simulink model "EnergyHub_V5_inf_buffer"  (R2024b)
settings: Solver=VariableStepAuto  StartTime=0  StopTime=31536000  MaxStep=1  RelTol=1e-3
values from neighbouring files (symbols this model uses):
  BatteryVNom = 51.2    [EdgeCases.m]    (also in MultipleModelTesting.m; setup_V3.m; setup_V5.m)
  ElectrolyserBoP = 80    [EdgeCases.m]    (also in setup_V3.m; setup_V5.m)
  ElectrolyserHoldTime = 25 * 60    (= 1500)    [EdgeCases.m]    (also in setup_V3.m; setup_V5.m)
  ElectrolyserHyFlow = 510    [EdgeCases.m]    (also in setup_V3.m; setup_V5.m)
  ElectrolyserPower = 2450    [EdgeCases.m]    (also in setup_V3.m = 2450/2:2450/2:2450*1.5; setup_V5.m)
  ElectrolyserRampDownTime = 30 * 60    (= 1800)    [EdgeCases.m]    (also in setup_V3.m; setup_V5.m)
  ElectrolyserRampUpTime = 10 * 60    (= 600)    [EdgeCases.m]    (also in setup_V3.m; setup_V5.m)
  ElectrolyserWarming = 260    [EdgeCases.m]    (also in setup_V3.m; setup_V5.m)
  ElectrolyserWarmingTime = 12 * 60    (= 720)    [EdgeCases.m]    (also in setup_V3.m; setup_V5.m)
  EMSElecStartHr = 14    [EdgeCases.m]    (also in setup_V3.m = 12:0.5:15; setup_V5.m)
  EMSElecStartSoC = 70    [EdgeCases.m]    (also in setup_V3.m = 70:5:80; setup_V5.m)
  EMSElecStopSoC = 65    [EdgeCases.m]    (also in setup_V3.m = 50:5:65; setup_V5.m)
  EMSFCSoCThresholds = [140, 150, 160, 170, 180]    [EdgeCases.m]    (also in setup_V3.m = [13, 14, 15, 16, 17]; setup_V5.m)
  EMSFCStartSoC = 15    [EdgeCases.m]    (also in MultipleModelTesting.m; setup_V3.m = 25; setup_V5.m)
  EMSFCStopSoC = 70    [EdgeCases.m]    (also in MultipleModelTesting.m; setup_V3.m = 90; setup_V5.m)
  EMSFCTimeThresholds = [113, 114, 115, 116, 117]    [EdgeCases.m]    (also in setup_V3.m = [40, 50, 60, 70, 80]; setup_V5.m)
  FuelCellAirBlower = 6.4*33.9    (= 216.96)    [EdgeCases.m]    (also in setup_V3.m; setup_V5.m)
  FuelCellBoP = 155    [EdgeCases.m]    (also in setup_V3.m; setup_V5.m)
  FuelCellHyFlow = 24    [EdgeCases.m]    (also in setup_V3.m = 31.7333333333; setup_V5.m)
  FuelCellPower = 2380    [EdgeCases.m]    (also in setup_V3.m = 1.2e3:300:1.8e3; setup_V5.m)
  FuelCellRampDown = 60    [EdgeCases.m]    (also in setup_V3.m; setup_V5.m)
  FuelCellRampTime1 = 40    [EdgeCases.m]    (also in setup_V3.m; setup_V5.m)
  FuelCellRampTime2 = 18*60    (= 1080)    [EdgeCases.m]    (also in setup_V3.m; setup_V5.m)
  FuelCellStartPower = 580    [EdgeCases.m]    (also in setup_V3.m; setup_V5.m)
  GridExtra = 0    [EdgeCases.m]    (also in setup_V3.m; setup_V5.m = 50)
  HydrogenCapacity = 70    [EdgeCases.m]    (also in setup_V3.m = 48; setup_V5.m)
  MinSoCGrid = EMSFCStartSoC-5    (= 10)    [EdgeCases.m]    (also in MultipleModelTesting.m; setup_V5.m)
  SolarPanels = 21    [EdgeCases.m]    (also in MultipleModelTesting.m = 12; setup_V3.m = 12:3:18; setup_V5.m = 18)
  SummerBase = 80    [EdgeCases.m]    (also in setup_V3.m; setup_V5.m)
  WinterBase = 235    [EdgeCases.m]    (also in setup_V3.m; setup_V5.m)
undefined symbols (not defined in the file or in its folder): Ion, Lithium
libraries: spsACVoltageSourceLib x3, spsBatteryLib x1, spsControlledCurrentSourceLib x1, sps_lib x1, simulink x1, spsGroundLib x1, spsPower3phInstantaneousLib x1, spsThreePhaseDynamicLoadLib x1, spsThreePhaseVIMeasurementLib x1
(part 1 of 2)
settings Model: Creator=daans  LastModifiedBy=daan
settings RTWCC: GPUComputeCapability=3.5

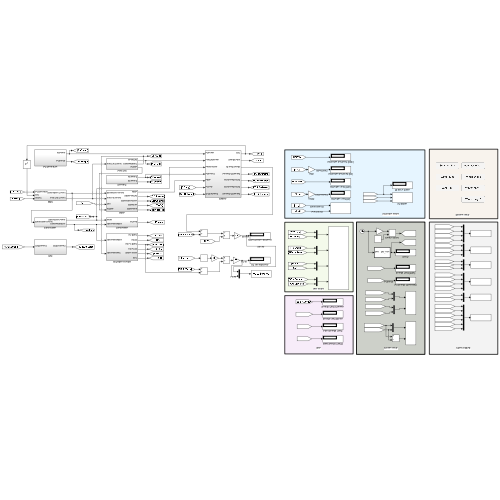
[thumbnail: Simulink's stored preview of the top-level diagram]
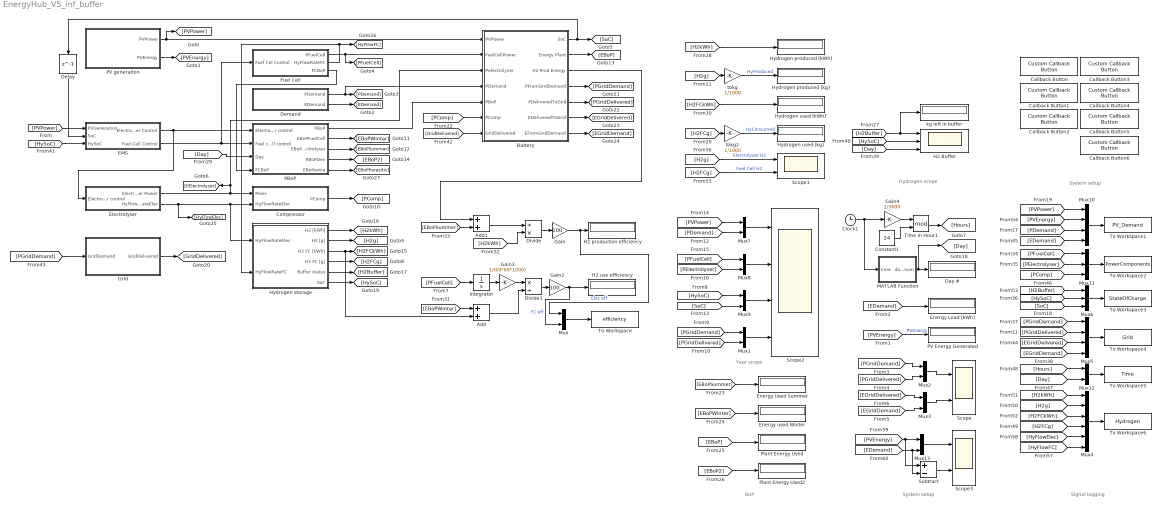
== system EnergyHub_V5_inf_buffer ==
  note: BoP
  note: System setup
  note: Year scope
  note: Hydrogen scope
  note: System setup
  note: Signal logging
  Add : Sum
  Add1 : Sum
  Battery : Subsystem
  Callback Button : CustomCallbackButton  Configuration="{\"components\":[{\"name\":\"BackgroundImageComponent\",\"settings\":{\"image\":{\"size\":[0,0],\"src\":\"default\",\"srcOrientation\":\"Right\"},\"position\":[0,0,1,1]}},{\"name\":\"ButtonStateComponent\",\"settings\":{\"buttonType\":\"momentary\",\"clickFcn\":\"% Define your start and stop time values\\nstartTime = 75*24*60*60;  % Example start time\\nstopTime = 289*24*60*60;   % Example stop time\\n\\n% Set the simulation start and stop time\\nset_param(gcs, 'StartTime', num2str(startTime));\\nset_param(gcs, 'StopTime', num2str(stopTime));\\n\\n% Optionally, start the simulation (if you want the button to trigger simulation)\\nset_param(gcs, 'SimulationCommand', 'start');\",\"onValue\":1,\"position\":[0,0,1,1],\"pressDelay\":\"500\",\"pressFcn\":\"\",\"repeatInterval\":\"0\",\"states\":[{\"horizontalAlignment\":\"center\",\"image\":{\"position\":[0,0,1,1],\"size\":[1,1],\"src\":\"default\",\"srcOrientation\":\"Right\"},\"label\":{\"color\":[0.01176470588,0.01176470588,0.01176470588,1],\"icon\":{\"size\":[0,0],\"src\":\"default\",\"srcOrientation\":\"Right\"},\"iconOffset\":0,\"iconPlacement\":\"left\",\"opacity\":1,\"show\":true,\"text\":{\"content\":\"Summer Sim\",\"font\":\"Helvetica\"}},\"labelOffset\":[0,0],\"verticalAlignment\":\"middle\"},{\"horizontalAlignment\":\"center\",\"image\":{\"position\":[0,0,1,1],\"size\":[1,1],\"src\":\"default\",\"srcOrientation\":\"Right\"},\"label\":{\"color\":[0.01176470588,0.01176470588,0.01176470588,1],\"icon\":{\"size\":[0,0],\"src\":\"default\",\"srcOrientation\":\"Right\"},\"iconOffset\":0,\"iconPlacement\":\"left\",\"opacity\":1,\"show\":true,\"text\":{\"content\":\"Summer Sim\",\"font\":\"Helvetica\"}},\"labelOffset\":[0,0],\"verticalAlignment\":\"middle\"},{\"horizontalAlignment\":\"center\",\"image\":{\"position\":[0,0,1,1],\"size\":[1,1],\"src\":\"default\",\"srcOrientation\":\"Right\"},\"label\":{\"color\":[0.01176470588,0.01176470588,0.01176470588,1],\"icon\":{\"size\":[0,0],\"src\":\"default\",\"srcOrientation\":\"Right\"},\"iconOffset\":0,\"iconPlacement\":\"left\",\"opacity\":1,\"show\":true,\"text\":{\"content\":\"Summer Sim\",\"font\":\"Helvetica\"}},\"labelOffset\":[0,0],\"verticalAlignment\":\"middle\"},{\"horizontalAlignment\":\"center\",\"image\":{\"position\":[0,0,1,1],\"size\":[1,1],\"src\":\"default\",\"srcOrientation\":\"Right\"},\"label\":{\"color\":[0.01176470588,0.01176470588,0.01176470588,1],\"icon\":{\"size\":[0,0],\"src\":\"default\",\"srcOrientation\":\"Right\"},\"iconOffset\":0,\"iconPlacement\":\"left\",\"opacity\":1,\"show\":true,\"text\":{\"content\":\"Summer Sim\",\"font\":\"Helvetica\"}},\"labelOffset\":[0,0],\"verticalAlignment\":\"middle\"}]}},{\"name\":\"ForegroundImageComponent\",\"settings\":{\"image\":{\"size\":[0,0],\"src\":\"default\",\"srcOrientation\":\"Right\"},\"isForeground\":1,\"position\":[0,0,1,1]}}],\"settings\":{\"BindingType\":\"standalone\",\"backgroundColor\":[244,244,244,1],\"backgroundOffset\":0.2,\"backgroundOpacity\":1,\"fixedAspectRatio\":\"off\",\"foregroundColor\":[0.01176470588,0.01176470588,0.01176470588,1],\"migratedFromLegacy\":true,\"useBackgroundColor\":true,\"variant\":\"callback\",\"version\":\"R2023a\"},\"type\":\"Button\"}"  CustomBackgroundColor="{\"color\":[0.9568627451,0.9568627451,0.9568627451],\"show\":true}"
  Callback Button1 : CustomCallbackButton  Configuration="{\"components\":[{\"name\":\"BackgroundImageComponent\",\"settings\":{\"image\":{\"size\":[0,0],\"src\":\"default\",\"srcOrientation\":\"Right\"},\"position\":[0,0,1,1]}},{\"name\":\"ButtonStateComponent\",\"settings\":{\"buttonType\":\"momentary\",\"clickFcn\":\"% Define your start and stop time values\\nstartTime = 19*24*60*60;  % Example start time\\nstopTime = 20*24*60*60;   % Example stop time\\n\\n% Set the simulation start and stop time\\nset_param(gcs, 'StartTime', num2str(startTime));\\nset_param(gcs, 'StopTime', num2str(stopTime));\\n\\n% Optionally, start the simulation (if you want the button to trigger simulation)\\nset_param(gcs, 'SimulationCommand', 'start');\",\"onValue\":1,\"position\":[0,0,1,1],\"pressDelay\":\"500\",\"pressFcn\":\"\",\"repeatInterval\":\"0\",\"states\":[{\"horizontalAlignment\":\"center\",\"image\":{\"position\":[0,0,1,1],\"size\":[1,1],\"src\":\"default\",\"srcOrientation\":\"Right\"},\"label\":{\"color\":[0.01176470588,0.01176470588,0.01176470588,1],\"icon\":{\"size\":[0,0],\"src\":\"default\",\"srcOrientation\":\"Right\"},\"iconOffset\":0,\"iconPlacement\":\"left\",\"opacity\":1,\"show\":true,\"text\":{\"content\":\"Winter Sim\",\"font\":\"Helvetica\"}},\"labelOffset\":[0,0],\"verticalAlignment\":\"middle\"},{\"horizontalAlignment\":\"center\",\"image\":{\"position\":[0,0,1,1],\"size\":[1,1],\"src\":\"default\",\"srcOrientation\":\"Right\"},\"label\":{\"color\":[0.01176470588,0.01176470588,0.01176470588,1],\"icon\":{\"size\":[0,0],\"src\":\"default\",\"srcOrientation\":\"Right\"},\"iconOffset\":0,\"iconPlacement\":\"left\",\"opacity\":1,\"show\":true,\"text\":{\"content\":\"Winter Sim\",\"font\":\"Helvetica\"}},\"labelOffset\":[0,0],\"verticalAlignment\":\"middle\"},{\"horizontalAlignment\":\"center\",\"image\":{\"position\":[0,0,1,1],\"size\":[1,1],\"src\":\"default\",\"srcOrientation\":\"Right\"},\"label\":{\"color\":[0.01176470588,0.01176470588,0.01176470588,1],\"icon\":{\"size\":[0,0],\"src\":\"default\",\"srcOrientation\":\"Right\"},\"iconOffset\":0,\"iconPlacement\":\"left\",\"opacity\":1,\"show\":true,\"text\":{\"content\":\"Winter Sim\",\"font\":\"Helvetica\"}},\"labelOffset\":[0,0],\"verticalAlignment\":\"middle\"},{\"horizontalAlignment\":\"center\",\"image\":{\"position\":[0,0,1,1],\"size\":[1,1],\"src\":\"default\",\"srcOrientation\":\"Right\"},\"label\":{\"color\":[0.01176470588,0.01176470588,0.01176470588,1],\"icon\":{\"size\":[0,0],\"src\":\"default\",\"srcOrientation\":\"Right\"},\"iconOffset\":0,\"iconPlacement\":\"left\",\"opacity\":1,\"show\":true,\"text\":{\"content\":\"Winter Sim\",\"font\":\"Helvetica\"}},\"labelOffset\":[0,0],\"verticalAlignment\":\"middle\"}]}},{\"name\":\"ForegroundImageComponent\",\"settings\":{\"image\":{\"size\":[0,0],\"src\":\"default\",\"srcOrientation\":\"Right\"},\"isForeground\":1,\"position\":[0,0,1,1]}}],\"settings\":{\"BindingType\":\"standalone\",\"backgroundColor\":[244,244,244,1],\"backgroundOffset\":0.2,\"backgroundOpacity\":1,\"fixedAspectRatio\":\"off\",\"foregroundColor\":[0.01176470588,0.01176470588,0.01176470588,1],\"migratedFromLegacy\":true,\"useBackgroundColor\":true,\"variant\":\"callback\",\"version\":\"R2023a\"},\"type\":\"Button\"}"  CustomBackgroundColor="{\"color\":[0.9568627451,0.9568627451,0.9568627451],\"show\":true}"
  Callback Button2 : CustomCallbackButton  Configuration="{\"components\":[{\"name\":\"BackgroundImageComponent\",\"settings\":{\"image\":{\"size\":[0,0],\"src\":\"default\",\"srcOrientation\":\"Right\"},\"position\":[0,0,1,1]}},{\"name\":\"ButtonStateComponent\",\"settings\":{\"buttonType\":\"momentary\",\"clickFcn\":\"% Define your start and stop time values\\nstartTime = 0;  % Example start time\\nstopTime = 365*24*60*60;   % Example stop time\\n\\n% Set the simulation start and stop time\\nset_param(gcs, 'StartTime', num2str(startTime));\\nset_param(gcs, 'StopTime', num2str(stopTime));\\n\\n% Optionally, start the simulation (if you want the button to trigger simulation)\\nset_param(gcs, 'SimulationCommand', 'start');\",\"onValue\":1,\"position\":[0,0,1,1],\"pressDelay\":\"500\",\"pressFcn\":\"\",\"repeatInterval\":\"0\",\"states\":[{\"horizontalAlignment\":\"center\",\"image\":{\"position\":[0,0,1,1],\"size\":[1,1],\"src\":\"default\",\"srcOrientation\":\"Right\"},\"label\":{\"color\":[0.01176470588,0.01176470588,0.01176470588,1],\"icon\":{\"size\":[0,0],\"src\":\"default\",\"srcOrientation\":\"Right\"},\"iconOffset\":0,\"iconPlacement\":\"left\",\"opacity\":1,\"show\":true,\"text\":{\"content\":\"Year Sim\",\"font\":\"Helvetica\"}},\"labelOffset\":[0,0],\"verticalAlignment\":\"middle\"},{\"horizontalAlignment\":\"center\",\"image\":{\"position\":[0,0,1,1],\"size\":[1,1],\"src\":\"default\",\"srcOrientation\":\"Right\"},\"label\":{\"color\":[0.01176470588,0.01176470588,0.01176470588,1],\"icon\":{\"size\":[0,0],\"src\":\"default\",\"srcOrientation\":\"Right\"},\"iconOffset\":0,\"iconPlacement\":\"left\",\"opacity\":1,\"show\":true,\"text\":{\"content\":\"Year Sim\",\"font\":\"Helvetica\"}},\"labelOffset\":[0,0],\"verticalAlignment\":\"middle\"},{\"horizontalAlignment\":\"center\",\"image\":{\"position\":[0,0,1,1],\"size\":[1,1],\"src\":\"default\",\"srcOrientation\":\"Right\"},\"label\":{\"color\":[0.01176470588,0.01176470588,0.01176470588,1],\"icon\":{\"size\":[0,0],\"src\":\"default\",\"srcOrientation\":\"Right\"},\"iconOffset\":0,\"iconPlacement\":\"left\",\"opacity\":1,\"show\":true,\"text\":{\"content\":\"Year Sim\",\"font\":\"Helvetica\"}},\"labelOffset\":[0,0],\"verticalAlignment\":\"middle\"},{\"horizontalAlignment\":\"center\",\"image\":{\"position\":[0,0,1,1],\"size\":[1,1],\"src\":\"default\",\"srcOrientation\":\"Right\"},\"label\":{\"color\":[0.01176470588,0.01176470588,0.01176470588,1],\"icon\":{\"size\":[0,0],\"src\":\"default\",\"srcOrientation\":\"Right\"},\"iconOffset\":0,\"iconPlacement\":\"left\",\"opacity\":1,\"show\":true,\"text\":{\"content\":\"Year Sim\",\"font\":\"Helvetica\"}},\"labelOffset\":[0,0],\"verticalAlignment\":\"middle\"}]}},{\"name\":\"ForegroundImageComponent\",\"settings\":{\"image\":{\"size\":[0,0],\"src\":\"default\",\"srcOrientation\":\"Right\"},\"isForeground\":1,\"position\":[0,0,1,1]}}],\"settings\":{\"BindingType\":\"standalone\",\"backgroundColor\":[244,244,244,1],\"backgroundOffset\":0.2,\"backgroundOpacity\":1,\"fixedAspectRatio\":\"off\",\"foregroundColor\":[0.01176470588,0.01176470588,0.01176470588,1],\"migratedFromLegacy\":true,\"useBackgroundColor\":true,\"variant\":\"callback\",\"version\":\"R2023a\"},\"type\":\"Button\"}"  CustomBackgroundColor="{\"color\":[0.9568627451,0.9568627451,0.9568627451],\"show\":true}"
  Callback Button3 : CustomCallbackButton  Configuration="{\"components\":[{\"name\":\"BackgroundImageComponent\",\"settings\":{\"image\":{\"size\":[0,0],\"src\":\"default\",\"srcOrientation\":\"Right\"},\"position\":[0,0,1,1]}},{\"name\":\"ButtonStateComponent\",\"settings\":{\"buttonType\":\"momentary\",\"clickFcn\":\"% Define your start and stop time values\\nstartTime = 166*24*60*60;  % Example start time\\nstopTime = 173*24*60*60;   % Example stop time\\n\\n% Set the simulation start and stop time\\nset_param(gcs, 'StartTime', num2str(startTime));\\nset_param(gcs, 'StopTime', num2str(stopTime));\\n\\n% Optionally, start the simulation (if you want the button to trigger simulation)\\nset_param(gcs, 'SimulationCommand', 'start');\",\"onValue\":1,\"position\":[0,0,1,1],\"pressDelay\":\"500\",\"pressFcn\":\"\",\"repeatInterval\":\"0\",\"states\":[{\"horizontalAlignment\":\"center\",\"image\":{\"position\":[0,0,1,1],\"size\":[1,1],\"src\":\"default\",\"srcOrientation\":\"Right\"},\"label\":{\"color\":[0.01176470588,0.01176470588,0.01176470588,1],\"icon\":{\"size\":[0,0],\"src\":\"default\",\"srcOrientation\":\"Right\"},\"iconOffset\":0,\"iconPlacement\":\"left\",\"opacity\":1,\"show\":true,\"text\":{\"content\":\"Summer Week\",\"font\":\"Helvetica\"}},\"labelOffset\":[0,0],\"verticalAlignment\":\"middle\"},{\"horizontalAlignment\":\"center\",\"image\":{\"position\":[0,0,1,1],\"size\":[1,1],\"src\":\"default\",\"srcOrientation\":\"Right\"},\"label\":{\"color\":[0.01176470588,0.01176470588,0.01176470588,1],\"icon\":{\"size\":[0,0],\"src\":\"default\",\"srcOrientation\":\"Right\"},\"iconOffset\":0,\"iconPlacement\":\"left\",\"opacity\":1,\"show\":true,\"text\":{\"content\":\"Summer Week\",\"font\":\"Helvetica\"}},\"labelOffset\":[0,0],\"verticalAlignment\":\"middle\"},{\"horizontalAlignment\":\"center\",\"image\":{\"position\":[0,0,1,1],\"size\":[1,1],\"src\":\"default\",\"srcOrientation\":\"Right\"},\"label\":{\"color\":[0.01176470588,0.01176470588,0.01176470588,1],\"icon\":{\"size\":[0,0],\"src\":\"default\",\"srcOrientation\":\"Right\"},\"iconOffset\":0,\"iconPlacement\":\"left\",\"opacity\":1,\"show\":true,\"text\":{\"content\":\"Summer Week\",\"font\":\"Helvetica\"}},\"labelOffset\":[0,0],\"verticalAlignment\":\"middle\"},{\"horizontalAlignment\":\"center\",\"image\":{\"position\":[0,0,1,1],\"size\":[1,1],\"src\":\"default\",\"srcOrientation\":\"Right\"},\"label\":{\"color\":[0.01176470588,0.01176470588,0.01176470588,1],\"icon\":{\"size\":[0,0],\"src\":\"default\",\"srcOrientation\":\"Right\"},\"iconOffset\":0,\"iconPlacement\":\"left\",\"opacity\":1,\"show\":true,\"text\":{\"content\":\"Summer Week\",\"font\":\"Helvetica\"}},\"labelOffset\":[0,0],\"verticalAlignment\":\"middle\"}]}},{\"name\":\"ForegroundImageComponent\",\"settings\":{\"image\":{\"size\":[0,0],\"src\":\"default\",\"srcOrientation\":\"Right\"},\"isForeground\":1,\"position\":[0,0,1,1]}}],\"settings\":{\"BindingType\":\"standalone\",\"backgroundColor\":[244,244,244,1],\"backgroundOffset\":0.2,\"backgroundOpacity\":1,\"fixedAspectRatio\":\"off\",\"foregroundColor\":[0.01176470588,0.01176470588,0.01176470588,1],\"migratedFromLegacy\":true,\"useBackgroundColor\":true,\"variant\":\"callback\",\"version\":\"R2023a\"},\"type\":\"Button\"}"  CustomBackgroundColor="{\"color\":[0.9568627451,0.9568627451,0.9568627451],\"show\":true}"
  Callback Button4 : CustomCallbackButton  Configuration="{\"components\":[{\"name\":\"BackgroundImageComponent\",\"settings\":{\"image\":{\"size\":[0,0],\"src\":\"default\",\"srcOrientation\":\"Right\"},\"position\":[0,0,1,1]}},{\"name\":\"ButtonStateComponent\",\"settings\":{\"buttonType\":\"momentary\",\"clickFcn\":\"% Define your start and stop time values\\nstartTime = 19*24*60*60;  % Example start time\\nstopTime = 26*24*60*60;   % Example stop time\\n\\n% Set the simulation start and stop time\\nset_param(gcs, 'StartTime', num2str(startTime));\\nset_param(gcs, 'StopTime', num2str(stopTime));\\n\\n% Optionally, start the simulation (if you want the button to trigger simulation)\\nset_param(gcs, 'SimulationCommand', 'start');\",\"onValue\":1,\"position\":[0,0,1,1],\"pressDelay\":\"500\",\"pressFcn\":\"\",\"repeatInterval\":\"0\",\"states\":[{\"horizontalAlignment\":\"center\",\"image\":{\"position\":[0,0,1,1],\"size\":[1,1],\"src\":\"default\",\"srcOrientation\":\"Right\"},\"label\":{\"color\":[0.01176470588,0.01176470588,0.01176470588,1],\"icon\":{\"size\":[0,0],\"src\":\"default\",\"srcOrientation\":\"Right\"},\"iconOffset\":0,\"iconPlacement\":\"left\",\"opacity\":1,\"show\":true,\"text\":{\"content\":\"Winter Week\",\"font\":\"Helvetica\"}},\"labelOffset\":[0,0],\"verticalAlignment\":\"middle\"},{\"horizontalAlignment\":\"center\",\"image\":{\"position\":[0,0,1,1],\"size\":[1,1],\"src\":\"default\",\"srcOrientation\":\"Right\"},\"label\":{\"color\":[0.01176470588,0.01176470588,0.01176470588,1],\"icon\":{\"size\":[0,0],\"src\":\"default\",\"srcOrientation\":\"Right\"},\"iconOffset\":0,\"iconPlacement\":\"left\",\"opacity\":1,\"show\":true,\"text\":{\"content\":\"Winter Week\",\"font\":\"Helvetica\"}},\"labelOffset\":[0,0],\"verticalAlignment\":\"middle\"},{\"horizontalAlignment\":\"center\",\"image\":{\"position\":[0,0,1,1],\"size\":[1,1],\"src\":\"default\",\"srcOrientation\":\"Right\"},\"label\":{\"color\":[0.01176470588,0.01176470588,0.01176470588,1],\"icon\":{\"size\":[0,0],\"src\":\"default\",\"srcOrientation\":\"Right\"},\"iconOffset\":0,\"iconPlacement\":\"left\",\"opacity\":1,\"show\":true,\"text\":{\"content\":\"Winter Week\",\"font\":\"Helvetica\"}},\"labelOffset\":[0,0],\"verticalAlignment\":\"middle\"},{\"horizontalAlignment\":\"center\",\"image\":{\"position\":[0,0,1,1],\"size\":[1,1],\"src\":\"default\",\"srcOrientation\":\"Right\"},\"label\":{\"color\":[0.01176470588,0.01176470588,0.01176470588,1],\"icon\":{\"size\":[0,0],\"src\":\"default\",\"srcOrientation\":\"Right\"},\"iconOffset\":0,\"iconPlacement\":\"left\",\"opacity\":1,\"show\":true,\"text\":{\"content\":\"Winter Week\",\"font\":\"Helvetica\"}},\"labelOffset\":[0,0],\"verticalAlignment\":\"middle\"}]}},{\"name\":\"ForegroundImageComponent\",\"settings\":{\"image\":{\"size\":[0,0],\"src\":\"default\",\"srcOrientation\":\"Right\"},\"isForeground\":1,\"position\":[0,0,1,1]}}],\"settings\":{\"BindingType\":\"standalone\",\"backgroundColor\":[244,244,244,1],\"backgroundOffset\":0.2,\"backgroundOpacity\":1,\"fixedAspectRatio\":\"off\",\"foregroundColor\":[0.01176470588,0.01176470588,0.01176470588,1],\"migratedFromLegacy\":true,\"useBackgroundColor\":true,\"variant\":\"callback\",\"version\":\"R2023a\"},\"type\":\"Button\"}"  CustomBackgroundColor="{\"color\":[0.9568627451,0.9568627451,0.9568627451],\"show\":true}"
  Callback Button5 : CustomCallbackButton  Configuration="{\"components\":[{\"name\":\"BackgroundImageComponent\",\"settings\":{\"image\":{\"size\":[0,0],\"src\":\"default\",\"srcOrientation\":\"Right\"},\"position\":[0,0,1,1]}},{\"name\":\"ButtonStateComponent\",\"settings\":{\"buttonType\":\"momentary\",\"clickFcn\":\"% Define your start and stop time values\\nstartTime = 0;  % Example start time\\nstopTime = 74*24*60*60;   % Example stop time\\n\\n% Set the simulation start and stop time\\nset_param(gcs, 'StartTime', num2str(startTime));\\nset_param(gcs, 'StopTime', num2str(stopTime));\\n\\n% Optionally, start the simulation (if you want the button to trigger simulation)\\nset_param(gcs, 'SimulationCommand', 'start');\",\"onValue\":1,\"position\":[0,0,1,1],\"pressDelay\":\"500\",\"pressFcn\":\"\",\"repeatInterval\":\"0\",\"states\":[{\"horizontalAlignment\":\"center\",\"image\":{\"position\":[0,0,1,1],\"size\":[1,1],\"src\":\"default\",\"srcOrientation\":\"Right\"},\"label\":{\"color\":[0.01176470588,0.01176470588,0.01176470588,1],\"icon\":{\"size\":[0,0],\"src\":\"default\",\"srcOrientation\":\"Right\"},\"iconOffset\":0,\"iconPlacement\":\"left\",\"opacity\":1,\"show\":true,\"text\":{\"content\":\"Winter only 1\",\"font\":\"Helvetica\"}},\"labelOffset\":[0,0],\"verticalAlignment\":\"middle\"},{\"horizontalAlignment\":\"center\",\"image\":{\"position\":[0,0,1,1],\"size\":[1,1],\"src\":\"default\",\"srcOrientation\":\"Right\"},\"label\":{\"color\":[0.01176470588,0.01176470588,0.01176470588,1],\"icon\":{\"size\":[0,0],\"src\":\"default\",\"srcOrientation\":\"Right\"},\"iconOffset\":0,\"iconPlacement\":\"left\",\"opacity\":1,\"show\":true,\"text\":{\"content\":\"Winter only 1\",\"font\":\"Helvetica\"}},\"labelOffset\":[0,0],\"verticalAlignment\":\"middle\"},{\"horizontalAlignment\":\"center\",\"image\":{\"position\":[0,0,1,1],\"size\":[1,1],\"src\":\"default\",\"srcOrientation\":\"Right\"},\"label\":{\"color\":[0.01176470588,0.01176470588,0.01176470588,1],\"icon\":{\"size\":[0,0],\"src\":\"default\",\"srcOrientation\":\"Right\"},\"iconOffset\":0,\"iconPlacement\":\"left\",\"opacity\":1,\"show\":true,\"text\":{\"content\":\"Winter only 1\",\"font\":\"Helvetica\"}},\"labelOffset\":[0,0],\"verticalAlignment\":\"middle\"},{\"horizontalAlignment\":\"center\",\"image\":{\"position\":[0,0,1,1],\"size\":[1,1],\"src\":\"default\",\"srcOrientation\":\"Right\"},\"label\":{\"color\":[0.01176470588,0.01176470588,0.01176470588,1],\"icon\":{\"size\":[0,0],\"src\":\"default\",\"srcOrientation\":\"Right\"},\"iconOffset\":0,\"iconPlacement\":\"left\",\"opacity\":1,\"show\":true,\"text\":{\"content\":\"Winter only 1\",\"font\":\"Helvetica\"}},\"labelOffset\":[0,0],\"verticalAlignment\":\"middle\"}]}},{\"name\":\"ForegroundImageComponent\",\"settings\":{\"image\":{\"size\":[0,0],\"src\":\"default\",\"srcOrientation\":\"Right\"},\"isForeground\":1,\"position\":[0,0,1,1]}}],\"settings\":{\"BindingType\":\"standalone\",\"backgroundColor\":[244,244,244,1],\"backgroundOffset\":0.2,\"backgroundOpacity\":1,\"fixedAspectRatio\":\"off\",\"foregroundColor\":[0.01176470588,0.01176470588,0.01176470588,1],\"migratedFromLegacy\":true,\"useBackgroundColor\":true,\"variant\":\"callback\",\"version\":\"R2023a\"},\"type\":\"Button\"}"  CustomBackgroundColor="{\"color\":[0.9568627451,0.9568627451,0.9568627451],\"show\":true}"
  Callback Button6 : CustomCallbackButton  Configuration="{\"components\":[{\"name\":\"BackgroundImageComponent\",\"settings\":{\"image\":{\"size\":[0,0],\"src\":\"default\",\"srcOrientation\":\"Right\"},\"position\":[0,0,1,1]}},{\"name\":\"ButtonStateComponent\",\"settings\":{\"buttonType\":\"momentary\",\"clickFcn\":\"% Define your start and stop time values\\nstartTime = 288*24*60*60;  % Example start time\\nstopTime = 365*24*60*60;   % Example stop time\\n\\n% Set the simulation start and stop time\\nset_param(gcs, 'StartTime', num2str(startTime));\\nset_param(gcs, 'StopTime', num2str(stopTime));\\n\\n% Optionally, start the simulation (if you want the button to trigger simulation)\\nset_param(gcs, 'SimulationCommand', 'start');\",\"onValue\":1,\"position\":[0,0,1,1],\"pressDelay\":\"500\",\"pressFcn\":\"\",\"repeatInterval\":\"0\",\"states\":[{\"horizontalAlignment\":\"center\",\"image\":{\"position\":[0,0,1,1],\"size\":[1,1],\"src\":\"default\",\"srcOrientation\":\"Right\"},\"label\":{\"color\":[0.01176470588,0.01176470588,0.01176470588,1],\"icon\":{\"size\":[0,0],\"src\":\"default\",\"srcOrientation\":\"Right\"},\"iconOffset\":0,\"iconPlacement\":\"left\",\"opacity\":1,\"show\":true,\"text\":{\"content\":\"Winter only 2\",\"font\":\"Helvetica\"}},\"labelOffset\":[0,0],\"verticalAlignment\":\"middle\"},{\"horizontalAlignment\":\"center\",\"image\":{\"position\":[0,0,1,1],\"size\":[1,1],\"src\":\"default\",\"srcOrientation\":\"Right\"},\"label\":{\"color\":[0.01176470588,0.01176470588,0.01176470588,1],\"icon\":{\"size\":[0,0],\"src\":\"default\",\"srcOrientation\":\"Right\"},\"iconOffset\":0,\"iconPlacement\":\"left\",\"opacity\":1,\"show\":true,\"text\":{\"content\":\"Winter only 2\",\"font\":\"Helvetica\"}},\"labelOffset\":[0,0],\"verticalAlignment\":\"middle\"},{\"horizontalAlignment\":\"center\",\"image\":{\"position\":[0,0,1,1],\"size\":[1,1],\"src\":\"default\",\"srcOrientation\":\"Right\"},\"label\":{\"color\":[0.01176470588,0.01176470588,0.01176470588,1],\"icon\":{\"size\":[0,0],\"src\":\"default\",\"srcOrientation\":\"Right\"},\"iconOffset\":0,\"iconPlacement\":\"left\",\"opacity\":1,\"show\":true,\"text\":{\"content\":\"Winter only 2\",\"font\":\"Helvetica\"}},\"labelOffset\":[0,0],\"verticalAlignment\":\"middle\"},{\"horizontalAlignment\":\"center\",\"image\":{\"position\":[0,0,1,1],\"size\":[1,1],\"src\":\"default\",\"srcOrientation\":\"Right\"},\"label\":{\"color\":[0.01176470588,0.01176470588,0.01176470588,1],\"icon\":{\"size\":[0,0],\"src\":\"default\",\"srcOrientation\":\"Right\"},\"iconOffset\":0,\"iconPlacement\":\"left\",\"opacity\":1,\"show\":true,\"text\":{\"content\":\"Winter only 2\",\"font\":\"Helvetica\"}},\"labelOffset\":[0,0],\"verticalAlignment\":\"middle\"}]}},{\"name\":\"ForegroundImageComponent\",\"settings\":{\"image\":{\"size\":[0,0],\"src\":\"default\",\"srcOrientation\":\"Right\"},\"isForeground\":1,\"position\":[0,0,1,1]}}],\"settings\":{\"BindingType\":\"standalone\",\"backgroundColor\":[244,244,244,1],\"backgroundOffset\":0.2,\"backgroundOpacity\":1,\"fixedAspectRatio\":\"off\",\"foregroundColor\":[0.01176470588,0.01176470588,0.01176470588,1],\"migratedFromLegacy\":true,\"useBackgroundColor\":true,\"variant\":\"callback\",\"version\":\"R2023a\"},\"type\":\"Button\"}"  CustomBackgroundColor="{\"color\":[0.9568627451,0.9568627451,0.9568627451],\"show\":true}"
  Clock1 : Clock
  Compressor : Subsystem
  Constant1 : Constant  Value=24
  Day # : Display
  Delay : Delay  DelayLength=1
  Demand : Subsystem
  Divide : Product  Inputs=/*
  Divide1 : Product  Inputs=*/
  EMS : Subsystem
  Electrolyser : Subsystem
  Energy Load [kWh] : Display
  Energy Used Summer : Display
  Energy used Winter : Display
  Fuel Cell : Subsystem
  Gain : Gain  Gain=100
  Gain2 : Gain  Gain=100
  Gain3 : Gain  Gain=1/(60*60*1000)
  Gain4 : Gain  Gain=1/3600
  Grid : Subsystem
  H2 Buffer : Scope  NumInputPorts=3
  H2 production efficiency : Display
  H2 use efficiency : Display
  Hydrogen produced [kWh] : Display
  Hydrogen produced [kg] : Display
  Hydrogen storage : Subsystem
  Hydrogen used [kWh] : Display
  Hydrogen used [kg] : Display
  Integrator : Integrator
  MATLAB Function : MATLAB Function  TreatAsAtomicUnit=on
  Mux{,1..3,7..9,12..13} (9 alike) : Mux  Inputs=2
  Mux10 : Mux
  Mux11 : Mux  Inputs=3
  Mux4 : Mux  Inputs=6
  Mux5 : Mux
  Mux6 : Mux  Inputs=3
  PBoP : Subsystem
  PV Energy Generated : Display
  PV generation : Subsystem
  Plant Energy Used : Display
  Plant Energy Used2 : Display
  Scope : Scope  NumInputPorts=2
  Scope1 : Scope  NumInputPorts=2
  Scope2 : Scope  NumInputPorts=4
  Scope3 : Scope  NumInputPorts=2
  Subtract : Sum  Inputs=+-
  Time in Hour1 : Math  Operator=mod
  To Workspace : ToWorkspace  VariableName=efficiency  SaveFormat=Timeseries  SampleTime=-1
      settings: Decimation=20
  To Workspace1 : ToWorkspace  VariableName=PV_Demand  SaveFormat=Timeseries  SampleTime=-1
      settings: Decimation=10
  To Workspace2 : ToWorkspace  VariableName=PowerComponents  SaveFormat=Timeseries  SampleTime=-1
  To Workspace3 : ToWorkspace  VariableName=StateOfCharge  SaveFormat=Timeseries  SampleTime=-1
      settings: Decimation=5
  To Workspace4 : ToWorkspace  VariableName=Grid  SaveFormat=Timeseries  SampleTime=-1
      settings: Decimation=10
  To Workspace5 : ToWorkspace  VariableName=Time  SaveFormat=Timeseries  SampleTime=-1
      settings: Decimation=20
  To Workspace6 : ToWorkspace  VariableName=Hydrogen  SaveFormat=Timeseries  SampleTime=-1
      settings: Decimation=10
  kg left in buffer : Display
  tokg : Gain  Gain=1/1000
  tokg2 : Gain  Gain=1/1000
  wires:
  PV generation/1(PVPower) -> Battery/1(PVPower), [PVPower]
  PV generation/2(PVEnergy) -> [PVEnergy]
  Electrolyser/1(Electrolyser Power) -> Battery/3(Pelectrolyser), [PElectrolyser], Compressor/1(Pelec)
  Electrolyser/2(HyFlowRateElec) -> Compressor/2(HyFlowRateElec), Hydrogen storage/1(HyFlowRateElec), [HyFlowElec]
  Hydrogen storage/2(H2 [g]) -> [H2g]
  Battery/2(Energy Plant) -> [EBoP]
  Divide/1 -> Gain/1
  Gain/1 -> Mux/1, H2 production efficiency/1  "Elec eff"
  Fuel Cell/1(PFuelCell) -> Battery/2(FuelCellPower), [PFuelCell]
  EMS/1(Electrolyser Control) -> PBoP/1(Electrolyser control), Electrolyser/1(Electrolyser control)
  Battery/1(SoC) -> [SoC], Delay/1
  [PVPower] -> EMS/1(PVGeneration)
  PBoP/1(PBoP) -> Battery/5(PBoP)
  EMS/2(Fuel Cell Control) -> Fuel Cell/1(Fuel Cel Control), PBoP/2(Fuel cell control)
  [PVEnergy] -> PV Energy Generated/1  "PVEnergy"
  Fuel Cell/2(HyFlowRateFC) -> Hydrogen storage/2(HyFlowRateFC), [HyFlowFC]
  [EDemand] -> Energy Load [kWh]/1
  Demand/2(EDemand) -> [EDemand]
  Hydrogen storage/1(H2 [kWh]) -> [H2kWh]
  Delay/1 -> EMS/2(SoC)
  Hydrogen storage/3(H2 FC [kWh]) -> [H2FCkWh], Add/2
  Gain2/1 -> Mux/2, H2 use efficiency/1  "FC eff"
  Divide1/1 -> Gain2/1
  [PFuelCell] -> Integrator/1
  Integrator/1 -> Gain3/1
  Gain3/1 -> Divide1/1
  Add1/1 -> Divide/1
  Add/1 -> Divide1/2
  Battery/3(H2 Prod Energy) -> Add1/1
  PBoP/3(EBoPElectrolyser) -> [EBoPSummer]
  PBoP/4(EBoPDev) -> [EBoP2]
  PBoP/2(EBoPFuelCell) -> [EBoPWinter]
  Gain4/1 -> Time in Hour1/1
  Constant1/1 -> Time in Hour1/2
  Time in Hour1/1 -> [Hours]
  Hydrogen storage/4(H2 FC [g]) -> [H2FCg]
  [PComp] -> Battery/6(PComp)
  [EBoPWinter] -> Energy used Winter/1
  [EBoPSummer] -> Energy Used Summer/1
  [EBoP] -> Plant Energy Used/1
  [EBoP2] -> Plant Energy Used2/1
  [H2FCkWh] -> Hydrogen used [kWh]/1
  [H2kWh] -> Hydrogen produced [kWh]/1
  Hydrogen storage/5(Buffer status) -> [H2Buffer]
  [H2Buffer] -> kg left in buffer/1, H2 Buffer/1
  Demand/1(PDemand) -> Battery/4(PDemand), [PDemand]
  Clock1/1 -> MATLAB Function/1(time), Gain4/1
  MATLAB Function/1(day_num) -> [Day], Day #/1
  [Day] -> PBoP/3(Day)
  [EBoPWinter] -> Add/1
  [H2kWh] -> Divide/2
  [EBoPSummer] -> Add1/2
  [H2g] -> tokg/1
  tokg/1 -> Hydrogen produced [kg]/1  "HyProduced"
  [H2FCg] -> tokg2/1
  tokg2/1 -> Hydrogen used [kg]/1  "HyConsumed"
  [PVPower] -> Mux7/1
  [PDemand] -> Mux7/2
  Mux7/1 -> Scope2/1
  Mux8/1 -> Scope2/2
  [PFuelCell] -> Mux8/1
  [PElectrolyser] -> Mux8/2
  [SoC] -> Mux9/2
  Mux9/1 -> Scope2/3
  Hydrogen storage/6(SoC) -> [HySoC]
  [HySoC] -> H2 Buffer/2
  [Day] -> H2 Buffer/3
  [HySoC] -> EMS/3(HySoC)
  [GridDelivered] -> Battery/7(GridDelivered)
  Grid/1(GridDelivered) -> [GridDelivered]
  [PGridDemand] -> Grid/1(GridDemand)
  Battery/4(PFromGridDemand) -> [PGridDemand]
  Battery/7(EFromGridDemand) -> [EGridDemand]
  Battery/6(EDeliveredToGrid) -> [EGridDelivered]
  Battery/5(PDeliveredToGrid) -> [PGridDelivered]
  [PGridDelivered] -> Mux2/2
  [PGridDemand] -> Mux2/1
  [EGridDelivered] -> Mux3/1
  [EGridDemand] -> Mux3/2
  Mux2/1 -> Scope/1
  Mux3/1 -> Scope/2
  [HySoC] -> Mux9/1
  Fuel Cell/3(FCBoP) -> PBoP/4(FCBoP)
  Mux1/1 -> Scope2/4
  [PGridDelivered] -> Mux1/2
  [PGridDemand] -> Mux1/1
  Compressor/1(PComp) -> [PComp]
  Mux/1 -> To Workspace/1
  [H2kWh] -> Mux4/1
  [H2g] -> Mux4/2
  [H2FCkWh] -> Mux4/3
  [H2FCg] -> Mux4/4
  [PGridDemand] -> Mux5/1
  [PGridDelivered] -> Mux5/2
  [EGridDelivered] -> Mux5/3
  [EGridDemand] -> Mux5/4
  [H2Buffer] -> Mux6/1
  [HySoC] -> Mux6/2
  [SoC] -> Mux6/3
  [PFuelCell] -> Mux11/1
  [PElectrolyser] -> Mux11/2
  [PComp] -> Mux11/3
  [PVPower] -> Mux10/1
  [PVEnergy] -> Mux10/2
  [PDemand] -> Mux10/3
  [EDemand] -> Mux10/4
  [Hours] -> Mux12/1
  [Day] -> Mux12/2
  Mux10/1 -> To Workspace1/1
  Mux11/1 -> To Workspace2/1
  Mux6/1 -> To Workspace3/1
  Mux5/1 -> To Workspace4/1
  Mux4/1 -> To Workspace6/1
  Mux12/1 -> To Workspace5/1
  [H2g] -> Scope1/1  "Electrolyser H2"
  [H2FCg] -> Scope1/2  "Fuel Cell H2"
  [HyFlowElec] -> Mux4/5
  [HyFlowFC] -> Mux4/6
  Mux13/1 -> Scope3/1
  [EDemand] -> Subtract/2, Mux13/2
  [PVEnergy] -> Subtract/1, Mux13/1
  Subtract/1 -> Scope3/2
  PBoP/5(EBoPextra) -> [EBoPParasitic]

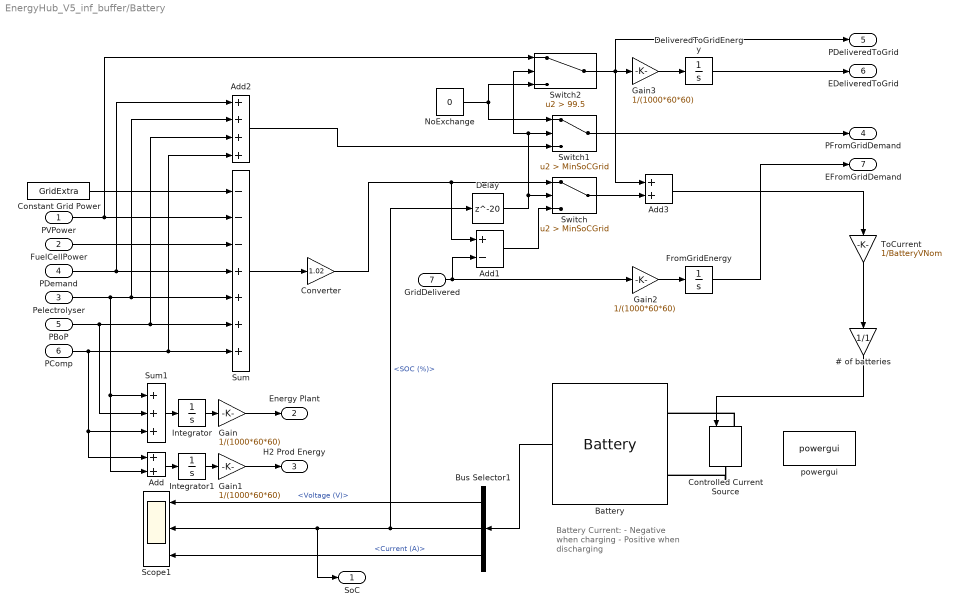
== system EnergyHub_V5_inf_buffer/Battery ==
  note: Battery Current:
      | - Negative when charging
      | - Positive when discharging
  PVPower : Inport
  FuelCellPower : Inport  Port=2
  Pelectrolyser : Inport  Port=3
  PDemand : Inport  Port=4
  PBoP : Inport  Port=5
  PComp : Inport  Port=6
  GridDelivered : Inport  Port=7
  "# of batteries " : Gain  Gain=1/1
  Add : Sum
  Add1 : Sum  Inputs=+-
  Add2 : Sum  Inputs=++++
  Add3 : Sum
  Battery : spsBatteryLib/Battery  BatType=Lithium-Ion  NomV=BatteryVNom  NomQ=BatteryCapacity  SOC=BatteryInitialSoC  Batt_Tr=1  PresetModel=on  MaxQ=300  MinV=38.4  FullV=59.5961  Dis_rate=130.4348  R=0.0017067  Normal_OP=271.3043  expZone="[55.3158      14.7391]"
      link override Model/Saturation: UpperLimit=95  LowerLimit=5
  Bus Selector1 : BusSelector  OutputSignals=Voltage (V),SOC (%),Current (A)
  Constant Grid Power : Constant  Value=GridExtra
  Controlled Current Source : spsControlledCurrentSourceLib/Controlled Current Source  Initialize=on  Source_Type=AC  Amplitude=0  Phase=0  Frequency=0  Measurements=None
  Converter : Gain  Gain=1.02
  Delay : Delay  DelayLength=20
  DeliveredToGridEnergy : Integrator
  FromGridEnergy : Integrator
  Gain{,1..3} (4 alike) : Gain  Gain=1/(1000*60*60)
  Integrator : Integrator
  Integrator1 : Integrator
  NoExchange : Constant  Value=0
  Scope1 : Scope  NumInputPorts=3
  Sum : Sum  Inputs=---++++
  Sum1 : Sum  Inputs=+++
  Switch : Switch  Criteria=u2 > Threshold  Threshold=MinSoCGrid  SaturateOnIntegerOverflow=off  InputSameDT=off
  Switch1 : Switch  Criteria=u2 > Threshold  Threshold=MinSoCGrid  SaturateOnIntegerOverflow=off  InputSameDT=off
  Switch2 : Switch  Criteria=u2 > Threshold  Threshold=99.5  SaturateOnIntegerOverflow=off  InputSameDT=off
  ToCurrent : Gain  Gain=1/BatteryVNom
  powergui : sps_lib/powergui  Priority=1  SimulationMode=Continuous  SampleTime=60  frequency=60  Iterations=50  frequencyindice=0  Pbase=100e6  ErrMax=1e-4  UnitsV=kV  UnitsW=MW  buscounter=0  FunctionMessages=off  echomessages=off  EnableUseOfTLC=off  CurrentSourceSwitches=off  DisableSnubberDevices=off  DisableRonSwitches=off  DisableVfSwitches=off  DisplayEquations=off  AutomaticDiscreteSolvers=off  SolverType=Tustin/Backward Euler (TBE)  Interpol=off  ExternalGateDelay=off  methode=off  Ts=100  x0status=blocks  SPID=on  SwTol=0  HookPort=off  NonlinearTolerance=1e-4  nMaxIteration=100  ContinueOnMaxIteration=off  RestoreLinks=warning  ResistiveCurrentMeasurement=off  Frange=[0:2:500]  Ylog=off  Xlog=on  ShowGrid=off  save=off  variable=ZData  structure=0  ZoomFFT=off  StartTime=0.0  cycles=1  DisplayStyle=1  fundamental=60  FreqAxis=off  MaxFrequency=1000  frequencyindicesteady=1  RmsSteady=1  display=off
  SoC : Outport
  Energy Plant : Outport  Port=2
  H2 Prod Energy : Outport  Port=3
  PFromGridDemand : Outport  Port=4
  PDeliveredToGrid : Outport  Port=5
  EDeliveredToGrid : Outport  Port=6
  EFromGridDemand : Outport  Port=7
  wires:
  ToCurrent/1 -> "# of batteries "/1
  Bus Selector1/3 -> Scope1/3  "<Current (A)>"
  Bus Selector1/2 -> SoC/1, Scope1/2, Delay/1  "<SOC (%)>"
  Bus Selector1/1 -> Scope1/1  "<Voltage (V)>"
  "# of batteries "/1 -> Controlled Current Source/1
  Battery/1 -> Bus Selector1/1
  PVPower/1 -> Sum/2, Switch2/1
  FuelCellPower/1 -> Sum/3
  PDemand/1 -> Add2/1, Sum/4
  Pelectrolyser/1 -> Add/2, Sum1/1, Add2/2, Sum/5
  PBoP/1 -> Sum1/2, Add2/3, Sum/6
  PComp/1 -> Add/1, Sum1/3, Sum/7, Add2/4
  Sum1/1 -> Integrator/1
  Integrator/1 -> Gain/1
  Gain/1 -> Energy Plant/1
  Sum/1 -> Converter/1
  Integrator1/1 -> Gain1/1
  Add/1 -> Integrator1/1
  Gain1/1 -> H2 Prod Energy/1
  Converter/1 -> Add1/1, Switch/1
  Add1/1 -> Switch/3
  Add2/1 -> Switch1/3
  Gain2/1 -> FromGridEnergy/1
  FromGridEnergy/1 -> EFromGridDemand/1
  Delay/1 -> Switch2/2, Switch1/2, Switch/2
  Switch1/1 -> PFromGridDemand/1
  NoExchange/1 -> Switch1/1, Switch2/3
  Constant Grid Power/1 -> Sum/1
  Switch2/1 -> Add3/1, PDeliveredToGrid/1, Gain3/1
  Gain3/1 -> DeliveredToGridEnergy/1
  DeliveredToGridEnergy/1 -> EDeliveredToGrid/1
  Add3/1 -> ToCurrent/1
  Switch/1 -> Add3/2
  GridDelivered/1 -> Gain2/1, Add1/2
  connections:
  Controlled Current Source/RConn1 -- Battery/LConn2
  Controlled Current Source/LConn1 -- Battery/LConn1

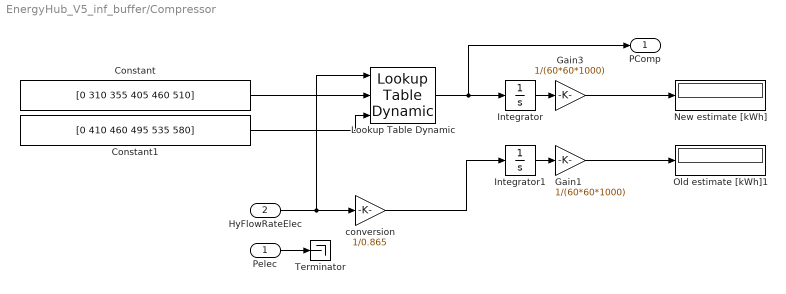
== system EnergyHub_V5_inf_buffer/Compressor ==
  Pelec : Inport
  HyFlowRateElec : Inport  Port=2
  Constant : Constant  Value=[0 310 355 405 460 510]
  Constant1 : Constant  Value=[0 410 460 495 535 580]
  Gain1 : Gain  Gain=1/(60*60*1000)
  Gain3 : Gain  Gain=1/(60*60*1000)
  Integrator : Integrator
  Integrator1 : Integrator
  Lookup Table Dynamic : simulink/Lookup Tables/Lookup Table Dynamic  LookUpMeth=Interpolation-Use End Values  OutDataType=fixdt('double')  OutScaling=[]  OutputDataTypeScalingMode=Specify via dialog  OutDataTypeStr=double  DoSatur=off
  New estimate [kWh] : Display
  Old estimate [kWh]1 : Display
  Terminator : Terminator
  conversion : Gain  Gain=1/0.865
  PComp : Outport
  wires:
  HyFlowRateElec/1 -> Lookup Table Dynamic/1, conversion/1
  Pelec/1 -> Terminator/1
  Lookup Table Dynamic/1 -> Integrator/1, PComp/1
  Integrator/1 -> Gain3/1
  Gain3/1 -> New estimate [kWh]/1
  Constant/1 -> Lookup Table Dynamic/2
  Constant1/1 -> Lookup Table Dynamic/3
  Integrator1/1 -> Gain1/1
  Gain1/1 -> Old estimate [kWh]1/1
  conversion/1 -> Integrator1/1

== system EnergyHub_V5_inf_buffer/Demand ==
  From Workspace : FromWorkspace  VariableName=PDemand
  Gain1 : Gain  Gain=1/(60*60*1000)
  Integrator : Integrator
  kW-to-W : Gain  Gain=1000
  PDemand : Outport
  EDemand : Outport  Port=2
  wires:
  From Workspace/1 -> kW-to-W/1
  kW-to-W/1 -> Integrator/1, PDemand/1
  Integrator/1 -> Gain1/1
  Gain1/1 -> EDemand/1

== system EnergyHub_V5_inf_buffer/EMS ==
  PVGeneration : Inport
  SoC : Inport  Port=2
  HySoC : Inport  Port=3
  Clock : Clock
  Electrolyser controller : Subsystem  mask{SoCmin=EMSElecStartSoC, TimeUntilStart=EMSElecStartHr, ShutDownSoC=EMSElecStopSoC}
      mask prompts: SoCmin "Min SoC: [%]"; TimeUntilStart "Time Until Start: [hr]"; ShutDownSoC "Shut down SoC: [%]"
  Subsystem : Subsystem  mask{START_SOC=EMSFCStartSoC, STOP_SOC=EMSFCStopSoC, SoCThresholds=EMSFCSoCThresholds, TimeThresholds=EMSFCTimeThresholds}
      mask prompts: START_SOC "Start FC SoC"; STOP_SOC "Stop FC SoC"; SoCThresholds "SoC thresholds"; TimeThresholds "Time thresholds"
  Electrolyser Control : Outport
  Fuel Cell Control : Outport  Port=2
  wires:
  SoC/1 -> Subsystem/1(Soc), Electrolyser controller/3(batterySoC)
  PVGeneration/1 -> Electrolyser controller/2(solarPower)
  Electrolyser controller/1(controlSignal) -> Electrolyser Control/1
  Clock/1 -> Electrolyser controller/1(timeInSeconds), Subsystem/2(time)
  Subsystem/1(FuelCellControl) -> Fuel Cell Control/1, Electrolyser controller/4(FCControl)
  HySoC/1 -> Subsystem/3(HySoC)

== system EnergyHub_V5_inf_buffer/Electrolyser ==
  Electrolyser control : Inport
  Clock : Clock
  MATLAB Function1 : MATLAB Function  Commented=on  TreatAsAtomicUnit=on
  Scope : Scope  NumInputPorts=2
  Subsystem : Subsystem  mask{ElectrolyserPower=ElectrolyserPower, ElectrolyserWarming=ElectrolyserWarming, ElectrolyserHyFlow=ElectrolyserHyFlow, ElectrolyserWarmingTime=ElectrolyserWarmingTime, ElectrolyserRampUpTime=ElectrolyserRampUpTime, ElectrolyserRampDownTime=ElectrolyserRampDownTime, ElectrolyserHoldTime=ElectrolyserHoldTime}
      mask prompts: ElectrolyserPower "Power Consumption: [W]"; ElectrolyserWarming "Warming Power Consumption: [W]"; ElectrolyserHyFlow "Max. Hydrogen flow rate: [NL/h]"; ElectrolyserWarmingTime "Warming up time: [s]"; ElectrolyserRampUpTime "Ramping up time: [s]"; ElectrolyserRampDownTime "Ramping down time: [s]"; ElectrolyserHoldTime "Hold time: [s]"
      mask DialogControl DescTextVar Prompt: Sub system mask for the electrolyser component. Inlude power consumption, max hydrogen flow rate, warming up power consumption, warming up time, ramping up time (60-100%), ramping down time (100-60%), and holding time.
  Electrolyser Power : Outport
  HyFlowRateElec : Outport  Port=2
  wires:
  Subsystem/1(ElectrolyserPower) -> Scope/1, Electrolyser Power/1
  Subsystem/2(HydrogenFlow) -> HyFlowRateElec/1, Scope/2
  Electrolyser control/1 -> Subsystem/1(controlLevel)
  Clock/1 -> Subsystem/2(time)

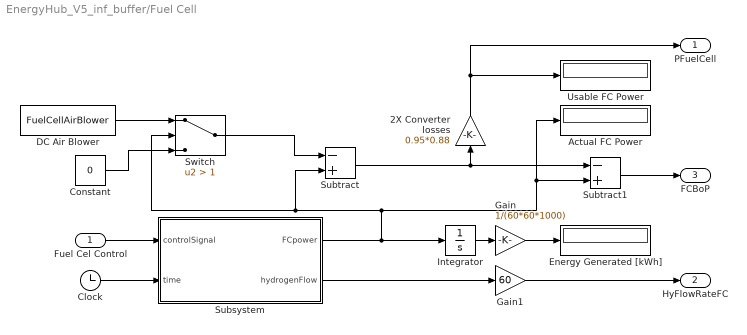
== system EnergyHub_V5_inf_buffer/Fuel Cell ==
  Fuel Cel Control : Inport
  2X Converter losses : Gain  Gain=0.95*0.88
  Actual FC Power : Display
  Clock : Clock
  Constant : Constant  Value=0
  DC Air Blower : Constant  Value=FuelCellAirBlower
  Energy Generated [kWh] : Display
  Gain : Gain  Gain=1/(60*60*1000)
  Gain1 : Gain  Gain=60
  Integrator : Integrator
  Subsystem : Subsystem  mask{FuelCellHyFlow=FuelCellHyFlow, FuelCellPower=FuelCellPower, FuelCellStartPower=FuelCellStartPower, FuelCellRampTime1=FuelCellRampTime1, FuelCellRampTime2=FuelCellRampTime2, FuelCellRampDown=FuelCellRampDown}
      mask prompts: FuelCellHyFlow "Fuel Cell Hydrogen Flow: [NL/min]"; FuelCellPower "Fuel Cell Power Genration: [W]"; FuelCellStartPower "Fuel Cell Start Power: [W]"; FuelCellRampTime1 "Fuel Cell Ramp Time (0 to start power): [s]"; FuelCellRampTime2 "Fuel Cell Ramp Time (start power to full power): [s]"; FuelCellRampDown "Fuel Cell Ramp Down Time (full power to 0): [s]"
      mask DialogControl DescTextVar Prompt: Sub system for the fuel cell component, including the parameters below.
  Subtract : Sum  Inputs=-+
  Subtract1 : Sum  Inputs=-+
  Switch : Switch  Criteria=u2 > Threshold  Threshold=1  SaturateOnIntegerOverflow=off  InputSameDT=off
  Usable FC Power : Display
  PFuelCell : Outport
  HyFlowRateFC : Outport  Port=2
  FCBoP : Outport  Port=3
  wires:
  Integrator/1 -> Gain/1
  Gain/1 -> Energy Generated [kWh]/1
  Gain1/1 -> HyFlowRateFC/1
  Subsystem/1(FCpower) -> Integrator/1, Actual FC Power/1, Subtract1/2, Subtract/2, Switch/2
  Fuel Cel Control/1 -> Subsystem/1(controlSignal)
  Clock/1 -> Subsystem/2(time)
  Subsystem/2(hydrogenFlow) -> Gain1/1
  Switch/1 -> Subtract/1
  DC Air Blower/1 -> Switch/1
  Constant/1 -> Switch/3
  Subtract1/1 -> FCBoP/1
  Subtract/1 -> 2X Converter losses/1, Subtract1/1
  2X Converter losses/1 -> PFuelCell/1, Usable FC Power/1

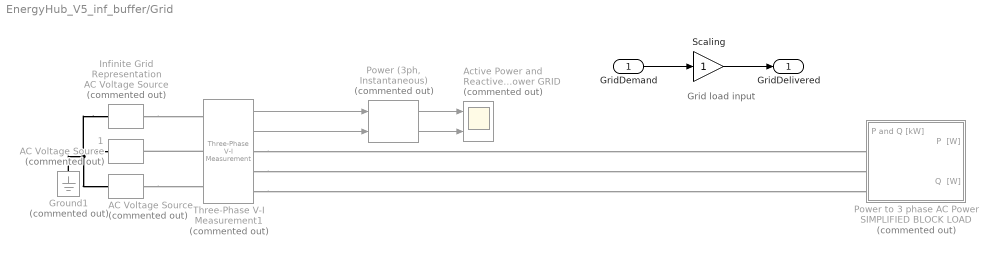
== system EnergyHub_V5_inf_buffer/Grid ==
  note: Grid
      | load input
  GridDemand : Inport
  " " : spsACVoltageSourceLib/AC Voltage Source  Commented=on  Amplitude=400*sqrt(2)  Phase=-240  Frequency=50  SampleTime=0  Measurements=None  BusType=swing  Pref=10e3  Qref=0  Qmin=-inf  Qmax=+inf
  "    1" : spsACVoltageSourceLib/AC Voltage Source  Commented=on  Amplitude=400*sqrt(2)  Phase=-120  Frequency=50  SampleTime=0  Measurements=None  BusType=swing  Pref=10e3  Qref=0  Qmin=-inf  Qmax=+inf
  "Active Power and Reactive Power GRID " : Scope  Commented=on  NumInputPorts=2
  Ground1 : spsGroundLib/Ground  Commented=on  LConnTagsString=a
  Infinite Grid Representation : spsACVoltageSourceLib/AC Voltage Source  Commented=on  Amplitude=400*sqrt(2)  Phase=0  Frequency=50  SampleTime=0  Measurements=None  BusType=swing  Pref=10e3  Qref=0  Qmin=-inf  Qmax=+inf
  "Power (3ph, Instantaneous)" : spsPower3phInstantaneousLib/Power (3ph, Instantaneous)  Commented=on
  Power to 3 phase AC Power SIMPLIFIED BLOCK LOAD : Subsystem  Commented=on
  Scaling : Gain
  Three-Phase V-I Measurement1 : spsThreePhaseVIMeasurementLib/Three-Phase V-I Measurement  Commented=on  VoltageMeasurement=phase-to-ground  SetLabelV=off  LabelV=Vabc  Vpu=off  VpuLL=off  CurrentMeasurement=yes  SetLabelI=off  LabelI=Iabc  Ipu=off  Pbase=100e6  Vbase=500e3  OutputType=Complex  PhasorSimulation=off  PSBequivalent=0
  GridDelivered : Outport
  wires:
  GridDemand/1 -> Scaling/1
  Three-Phase V-I Measurement1/1 -> "Power (3ph, Instantaneous)"/1
  "Power (3ph, Instantaneous)"/1 -> "Active Power and Reactive Power GRID "/1
  "Power (3ph, Instantaneous)"/2 -> "Active Power and Reactive Power GRID "/2
  Three-Phase V-I Measurement1/2 -> "Power (3ph, Instantaneous)"/2
  Scaling/1 -> GridDelivered/1
  connections:
  Infinite Grid Representation/RConn1 -- Three-Phase V-I Measurement1/LConn1
  Three-Phase V-I Measurement1/LConn2 -- "    1"/RConn1
  " "/RConn1 -- Three-Phase V-I Measurement1/LConn3
  Infinite Grid Representation/LConn1 -- Ground1/LConn1 -- " "/LConn1 -- "    1"/LConn1
  Three-Phase V-I Measurement1/RConn2 -- Power to 3 phase AC Power SIMPLIFIED BLOCK LOAD/LConn2
  Three-Phase V-I Measurement1/RConn1 -- Power to 3 phase AC Power SIMPLIFIED BLOCK LOAD/LConn1
  Three-Phase V-I Measurement1/RConn3 -- Power to 3 phase AC Power SIMPLIFIED BLOCK LOAD/LConn3

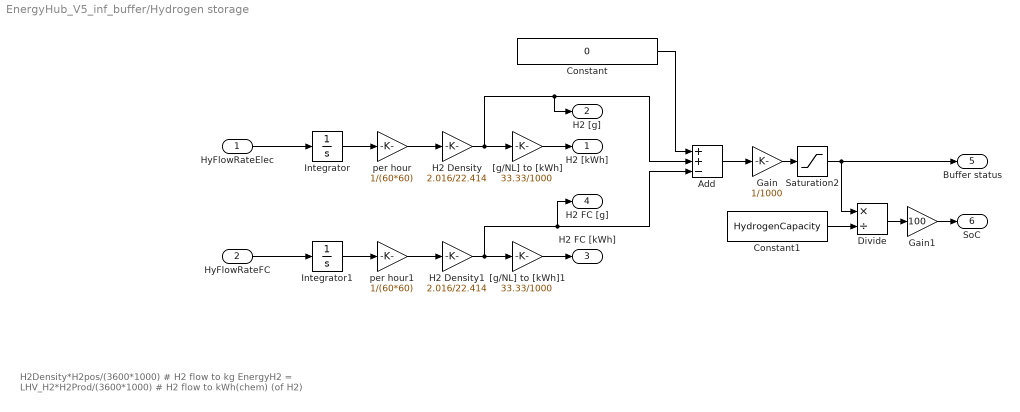
== system EnergyHub_V5_inf_buffer/Hydrogen storage ==
  note: H2Density*H2pos/(3600*1000) # H2 flow to kg
      | EnergyH2 = LHV_H2*H2Prod/(3600*1000) # H2 flow to kWh(chem) (of H2)
  HyFlowRateElec : Inport
  HyFlowRateFC : Inport  Port=2
  Add : Sum  Inputs=++-
  Constant : Constant  Value=0
  Constant1 : Constant  Value=HydrogenCapacity
  Divide : Product  Inputs=*/
  Gain : Gain  Gain=1/1000
  Gain1 : Gain  Gain=100
  H2 Density : Gain  Gain=2.016/22.414
  H2 Density1 : Gain  Gain=2.016/22.414
  Integrator : Integrator
  Integrator1 : Integrator
  Saturation2 : Saturate  UpperLimit=1000  LowerLimit=-1000
  "[g/NL] to [kWh]" : Gain  Gain=33.33/1000
  "[g/NL] to [kWh]1" : Gain  Gain=33.33/1000
  per hour : Gain  Gain=1/(60*60)
  per hour1 : Gain  Gain=1/(60*60)
  H2 [kWh] : Outport
  H2 [g] : Outport  Port=2
  H2 FC [kWh] : Outport  Port=3
  H2 FC [g] : Outport  Port=4
  Buffer status : Outport  Port=5
  SoC : Outport  Port=6
  wires:
  HyFlowRateElec/1 -> Integrator/1
  Integrator/1 -> per hour/1
  "[g/NL] to [kWh]"/1 -> H2 [kWh]/1
  per hour/1 -> H2 Density/1
  H2 Density/1 -> H2 [g]/1, Add/2, "[g/NL] to [kWh]"/1
  "[g/NL] to [kWh]1"/1 -> H2 FC [kWh]/1
  per hour1/1 -> H2 Density1/1
  H2 Density1/1 -> Add/3, H2 FC [g]/1, "[g/NL] to [kWh]1"/1
  HyFlowRateFC/1 -> Integrator1/1
  Integrator1/1 -> per hour1/1
  Constant/1 -> Add/1
  Constant1/1 -> Divide/2
  Divide/1 -> Gain1/1
  Gain1/1 -> SoC/1
  Add/1 -> Gain/1
  Gain/1 -> Saturation2/1
  Saturation2/1 -> Divide/1, Buffer status/1
